simulink model "HVDC_VSC_1CPUcore_dcpl"  (Simulink 8.4)
settings: Solver=ode3  SolverMode=SingleTasking  StartTime=0.0  StopTime=70.0  FixedStep=Ts_Power  RelTol=1e-3  AbsTol=1e-2
PreLoadFcn:
  | Ts_Power=50e-6; Ts_Control=1*Ts_Power; init_cosim_IA; startup_transients_hvdc_vsc;
PostLoadFcn:
  | Ts_Power=50e-6; Ts_Control=1*Ts_Power; init_cosim_IA; startup_transients_hvdc_vsc;
InitFcn:
  | Ts_Power=50e-6; Ts_Control=1*Ts_Power; init_cosim_IA; startup_transients_hvdc_vsc;
values from neighbouring files (symbols this model uses):
  dPref1_2 = 0.125    [startup_transients_hvdc_vsc.m]
  dPref1_2_rlimit = 0.6    [startup_transients_hvdc_vsc.m]
  t_deblock_Pref1 = 0.5    [startup_transients_hvdc_vsc.m]
  t_deblock_Udref2 = 0.3    [startup_transients_hvdc_vsc.m]
  t_dPref1_2 = 25.0    (= 25)    [startup_transients_hvdc_vsc.m]
  t_SwitchITMIdc = 0.2    [startup_transients_hvdc_vsc.m]
  t_SwitchITMVdc = 0.1    [startup_transients_hvdc_vsc.m]
undefined symbols (not defined in the file or in its folder): CLARK, D1, Delta, gcbh, h, intfDelay, level, lib_mesures, magnitude, ResistanceM, rte_drive_private_lib, rte_tsb3level_hiz_rect_cb, sps_rtmsupport, Ts_intf, TSB3_hiZR
libraries: powerlib x183, spsVIMeasurementModel x102, powerlib_extras x71, powerlib_meascontrol x50, rteventslib x26, op_dpl_lib x20, rtlab x12, sps_avr x6, artemis x1
(part 6 of 13)

== system HVDC_VSC_1CPUcore_dcpl/SM_HVDC_VSC/37.5-km  cable1/Artemis DPL2 ==
  hi : Inport
  GroundI_0_1 : powerlib/Elements/Ground  LConnTagsString=a
  GroundR_0_1 : powerlib/Elements/Ground  LConnTagsString=a
  ISource_0_1 : powerlib/Electrical Sources/Controlled Current Source  Initialize=off  Source_Type=AC  Amplitude=0  Phase=0  Frequency=0  Measurements=None
  R_0_1 : powerlib/Elements/Series RLC Branch  LConnTagsString=__new0  RConnTagsString=__new0  BranchType=R  Resistance=ResistanceM(1,1)  Inductance=1.0  SetiL0=off  InitialCurrent=0  Capacitance=1.0  Setx0=off  InitialVoltage=0  Measurements=None
  VMeasure_0_1 : powerlib/Measurements/Voltage Measurement  PhasorSimulation=off  OutputType=Complex  PSBequivalent=0
  separated_model1 : op_dpl_lib/separated_model1  nphase=Phases  f=Frequency  ri=Resistance  li=Inductance  ci=Capacitance  long=Length  V1_init=[0 zeros(1,Phases); 0.1 zeros(1,Phases)]  V2_init=[0 zeros(1,Phases); 0.1 zeros(1,Phases)]  I1_init=[0 zeros(1,Phases); 0.1 zeros(1,Phases)]  I2_init=[0 zeros(1,Phases); 0.1 zeros(1,Phases)]  time_init=0.000622095723695317
  PM1 : PMIOPort  Port=1  Side=Left
  ho : Outport
  wires:
  [ho] -> ho/1
  hi/1 -> [hi]
  [V_A_1] -> separated_model1/1
  separated_model1/1 -> [I_A_1]
  [hi] -> separated_model1/2
  separated_model1/2 -> [ho]
  [I_A_1] -> ISource_0_1/1
  VMeasure_0_1/1 -> [V_A_1]
  connections:
  VMeasure_0_1/LConn1 -- ISource_0_1/RConn1 -- R_0_1/LConn1 -- PM1/RConn1
  VMeasure_0_1/LConn2 -- GroundI_0_1/LConn1 -- ISource_0_1/LConn1
  R_0_1/RConn1 -- GroundR_0_1/LConn1

== system HVDC_VSC_1CPUcore_dcpl/SM_HVDC_VSC/37.5-km  cable1/BI ==

== system HVDC_VSC_1CPUcore_dcpl/SM_HVDC_VSC/37.5-km cable/Artemis DPL1 ==
  hi : Inport
  GroundI_0_1 : powerlib/Elements/Ground  LConnTagsString=a
  GroundR_0_1 : powerlib/Elements/Ground  LConnTagsString=a
  ISource_0_1 : powerlib/Electrical Sources/Controlled Current Source  Initialize=off  Source_Type=AC  Amplitude=0  Phase=0  Frequency=0  Measurements=None
  R_0_1 : powerlib/Elements/Series RLC Branch  LConnTagsString=__new0  RConnTagsString=__new0  BranchType=R  Resistance=ResistanceM(1,1)  Inductance=1.0  SetiL0=off  InitialCurrent=0  Capacitance=1.0  Setx0=off  InitialVoltage=0  Measurements=None
  VMeasure_0_1 : powerlib/Measurements/Voltage Measurement  PhasorSimulation=off  OutputType=Complex  PSBequivalent=0
  separated_model1 : op_dpl_lib/separated_model1  nphase=Phases  f=Frequency  ri=Resistance  li=Inductance  ci=Capacitance  long=Length  V1_init=[0 zeros(1,Phases); 0.1 zeros(1,Phases)]  V2_init=[0 zeros(1,Phases); 0.1 zeros(1,Phases)]  I1_init=[0 zeros(1,Phases); 0.1 zeros(1,Phases)]  I2_init=[0 zeros(1,Phases); 0.1 zeros(1,Phases)]  time_init=0.000622095723695317
  PM1 : PMIOPort  Port=1  Side=Left
  ho : Outport
  wires:
  [ho] -> ho/1
  hi/1 -> [hi]
  [V_A_1] -> separated_model1/1
  separated_model1/1 -> [I_A_1]
  [hi] -> separated_model1/2
  separated_model1/2 -> [ho]
  [I_A_1] -> ISource_0_1/1
  VMeasure_0_1/1 -> [V_A_1]
  connections:
  VMeasure_0_1/LConn1 -- ISource_0_1/RConn1 -- R_0_1/LConn1 -- PM1/RConn1
  VMeasure_0_1/LConn2 -- GroundI_0_1/LConn1 -- ISource_0_1/LConn1
  R_0_1/RConn1 -- GroundR_0_1/LConn1

== system HVDC_VSC_1CPUcore_dcpl/SM_HVDC_VSC/37.5-km cable/Artemis DPL2 ==
  hi : Inport
  GroundI_0_1 : powerlib/Elements/Ground  LConnTagsString=a
  GroundR_0_1 : powerlib/Elements/Ground  LConnTagsString=a
  ISource_0_1 : powerlib/Electrical Sources/Controlled Current Source  Initialize=off  Source_Type=AC  Amplitude=0  Phase=0  Frequency=0  Measurements=None
  R_0_1 : powerlib/Elements/Series RLC Branch  LConnTagsString=__new0  RConnTagsString=__new0  BranchType=R  Resistance=ResistanceM(1,1)  Inductance=1.0  SetiL0=off  InitialCurrent=0  Capacitance=1.0  Setx0=off  InitialVoltage=0  Measurements=None
  VMeasure_0_1 : powerlib/Measurements/Voltage Measurement  PhasorSimulation=off  OutputType=Complex  PSBequivalent=0
  separated_model1 : op_dpl_lib/separated_model1  nphase=Phases  f=Frequency  ri=Resistance  li=Inductance  ci=Capacitance  long=Length  V1_init=[0 zeros(1,Phases); 0.1 zeros(1,Phases)]  V2_init=[0 zeros(1,Phases); 0.1 zeros(1,Phases)]  I1_init=[0 zeros(1,Phases); 0.1 zeros(1,Phases)]  I2_init=[0 zeros(1,Phases); 0.1 zeros(1,Phases)]  time_init=0.000622095723695317
  PM1 : PMIOPort  Port=1  Side=Left
  ho : Outport
  wires:
  [ho] -> ho/1
  hi/1 -> [hi]
  [V_A_1] -> separated_model1/1
  separated_model1/1 -> [I_A_1]
  [hi] -> separated_model1/2
  separated_model1/2 -> [ho]
  [I_A_1] -> ISource_0_1/1
  VMeasure_0_1/1 -> [V_A_1]
  connections:
  VMeasure_0_1/LConn1 -- ISource_0_1/RConn1 -- R_0_1/LConn1 -- PM1/RConn1
  VMeasure_0_1/LConn2 -- GroundI_0_1/LConn1 -- ISource_0_1/LConn1
  R_0_1/RConn1 -- GroundR_0_1/LConn1

== system HVDC_VSC_1CPUcore_dcpl/SM_HVDC_VSC/37.5-km cable/BI ==

== system HVDC_VSC_1CPUcore_dcpl/SM_HVDC_VSC/37.5-km cable1/Artemis DPL1 ==
  hi : Inport
  GroundI_0_1 : powerlib/Elements/Ground  LConnTagsString=a
  GroundR_0_1 : powerlib/Elements/Ground  LConnTagsString=a
  ISource_0_1 : powerlib/Electrical Sources/Controlled Current Source  Initialize=off  Source_Type=AC  Amplitude=0  Phase=0  Frequency=0  Measurements=None
  R_0_1 : powerlib/Elements/Series RLC Branch  LConnTagsString=__new0  RConnTagsString=__new0  BranchType=R  Resistance=ResistanceM(1,1)  Inductance=1.0  SetiL0=off  InitialCurrent=0  Capacitance=1.0  Setx0=off  InitialVoltage=0  Measurements=None
  VMeasure_0_1 : powerlib/Measurements/Voltage Measurement  PhasorSimulation=off  OutputType=Complex  PSBequivalent=0
  separated_model1 : op_dpl_lib/separated_model1  nphase=Phases  f=Frequency  ri=Resistance  li=Inductance  ci=Capacitance  long=Length  V1_init=[0 zeros(1,Phases); 0.1 zeros(1,Phases)]  V2_init=[0 zeros(1,Phases); 0.1 zeros(1,Phases)]  I1_init=[0 zeros(1,Phases); 0.1 zeros(1,Phases)]  I2_init=[0 zeros(1,Phases); 0.1 zeros(1,Phases)]  time_init=0.000622095723695317
  PM1 : PMIOPort  Port=1  Side=Left
  ho : Outport
  wires:
  VMeasure_0_1/1 -> [V_A_1]
  [I_A_1] -> ISource_0_1/1
  separated_model1/2 -> [ho]
  [hi] -> separated_model1/2
  separated_model1/1 -> [I_A_1]
  [V_A_1] -> separated_model1/1
  hi/1 -> [hi]
  [ho] -> ho/1
  connections:
  R_0_1/RConn1 -- GroundR_0_1/LConn1
  ISource_0_1/LConn1 -- GroundI_0_1/LConn1 -- VMeasure_0_1/LConn2
  PM1/RConn1 -- R_0_1/LConn1 -- ISource_0_1/RConn1 -- VMeasure_0_1/LConn1

== system HVDC_VSC_1CPUcore_dcpl/SM_HVDC_VSC/37.5-km cable1/Artemis DPL2 ==
  hi : Inport
  GroundI_0_1 : powerlib/Elements/Ground  LConnTagsString=a
  GroundR_0_1 : powerlib/Elements/Ground  LConnTagsString=a
  ISource_0_1 : powerlib/Electrical Sources/Controlled Current Source  Initialize=off  Source_Type=AC  Amplitude=0  Phase=0  Frequency=0  Measurements=None
  R_0_1 : powerlib/Elements/Series RLC Branch  LConnTagsString=__new0  RConnTagsString=__new0  BranchType=R  Resistance=ResistanceM(1,1)  Inductance=1.0  SetiL0=off  InitialCurrent=0  Capacitance=1.0  Setx0=off  InitialVoltage=0  Measurements=None
  VMeasure_0_1 : powerlib/Measurements/Voltage Measurement  PhasorSimulation=off  OutputType=Complex  PSBequivalent=0
  separated_model1 : op_dpl_lib/separated_model1  nphase=Phases  f=Frequency  ri=Resistance  li=Inductance  ci=Capacitance  long=Length  V1_init=[0 zeros(1,Phases); 0.1 zeros(1,Phases)]  V2_init=[0 zeros(1,Phases); 0.1 zeros(1,Phases)]  I1_init=[0 zeros(1,Phases); 0.1 zeros(1,Phases)]  I2_init=[0 zeros(1,Phases); 0.1 zeros(1,Phases)]  time_init=0.000622095723695317
  PM1 : PMIOPort  Port=1  Side=Left
  ho : Outport
  wires:
  VMeasure_0_1/1 -> [V_A_1]
  [I_A_1] -> ISource_0_1/1
  separated_model1/2 -> [ho]
  [hi] -> separated_model1/2
  separated_model1/1 -> [I_A_1]
  [V_A_1] -> separated_model1/1
  hi/1 -> [hi]
  [ho] -> ho/1
  connections:
  R_0_1/RConn1 -- GroundR_0_1/LConn1
  ISource_0_1/LConn1 -- GroundI_0_1/LConn1 -- VMeasure_0_1/LConn2
  PM1/RConn1 -- R_0_1/LConn1 -- ISource_0_1/RConn1 -- VMeasure_0_1/LConn1

== system HVDC_VSC_1CPUcore_dcpl/SM_HVDC_VSC/37.5-km cable1/BI ==

== system HVDC_VSC_1CPUcore_dcpl/SM_HVDC_VSC/Station 1 (Rectifier)/Bconv1 ==
  Kv : Gain  Gain=Ki  SaturateOnIntegerOverflow=on  OutDataTypeStr=Inherit: Same as input  ParamDataTypeStr=Inherit: Same as input
  Kv1 : Gain  Gain=Kv  SaturateOnIntegerOverflow=on  OutDataTypeStr=Inherit: Same as input  ParamDataTypeStr=Inherit: Same as input
  Mode I : spsVIMeasurementModel/Complex
  Mode V : spsVIMeasurementModel/Complex
  Model : spsVIMeasurementModel/VI  SystemSampleTime=-1
  A : PMIOPort  Port=1  Side=Left
  B : PMIOPort  Port=2  Side=Left
  C : PMIOPort  Port=3  Side=Left
  a : PMIOPort  Port=4  Side=Right
  b : PMIOPort  Port=5  Side=Right
  c : PMIOPort  Port=6  Side=Right
  tag scope: Iv_abc1=global, Uv_abc1=global
  wires:
  Model/2 -> Kv/1
  Model/1 -> Kv1/1
  Kv/1 -> Mode I/1
  Kv1/1 -> Mode V/1
  Mode I/1 -> [Iv_abc1]
  Mode V/1 -> [Uv_abc1]
  connections:
  Model/RConn3 -- c/RConn1
  Model/RConn1 -- a/RConn1
  Model/RConn2 -- b/RConn1
  Model/LConn3 -- C/RConn1
  Model/LConn1 -- A/RConn1
  Model/LConn2 -- B/RConn1

== system HVDC_VSC_1CPUcore_dcpl/SM_HVDC_VSC/Station 1 (Rectifier)/Bfilter1 ==
  Iabc : Terminator
  Kv : Gain  Gain=Ki  SaturateOnIntegerOverflow=on  OutDataTypeStr=Inherit: Same as input  ParamDataTypeStr=Inherit: Same as input
  Kv1 : Gain  Gain=Kv  SaturateOnIntegerOverflow=on  OutDataTypeStr=Inherit: Same as input  ParamDataTypeStr=Inherit: Same as input
  Mode I : spsVIMeasurementModel/Complex
  Mode V : spsVIMeasurementModel/Complex
  Model : spsVIMeasurementModel/V  SystemSampleTime=-1
  A : PMIOPort  Port=1  Side=Left
  B : PMIOPort  Port=2  Side=Left
  C : PMIOPort  Port=3  Side=Left
  a : PMIOPort  Port=4  Side=Right
  b : PMIOPort  Port=5  Side=Right
  c : PMIOPort  Port=6  Side=Right
  tag scope: Uf_abc1=global
  wires:
  Model/2 -> Kv/1
  Model/1 -> Kv1/1
  Kv/1 -> Mode I/1
  Kv1/1 -> Mode V/1
  Mode I/1 -> Iabc/1
  Mode V/1 -> [Uf_abc1]
  connections:
  Model/RConn3 -- c/RConn1
  Model/RConn1 -- a/RConn1
  Model/RConn2 -- b/RConn1
  Model/LConn3 -- C/RConn1
  Model/LConn1 -- A/RConn1
  Model/LConn2 -- B/RConn1

== system HVDC_VSC_1CPUcore_dcpl/SM_HVDC_VSC/Station 1 (Rectifier)/Filters 60Hz2 ==
  note: High-pass
      | damped filters
  note: AC Filters, 40 Mvar @ 100 kV
  "27th 18 Mvar Q = 15 " : powerlib/Elements/Three-Phase Harmonic Filter  LConnTagsString=A|B|C  FilterType=High-pass  FilterConnection=Y (grounded)  ParNom="[100e3  60]"  Qc=80e6 * 0.45  Fr=27*60  Frd=[11*60 13*60]  Q=15  Measurements=None
      settings: AttributesFormatString=\n
  "54th 22 Mvar Q = 15 " : powerlib/Elements/Three-Phase Harmonic Filter  LConnTagsString=A|B|C  FilterType=High-pass  FilterConnection=Y (grounded)  ParNom="[100e3  60]"  Qc=80e6 * 0.55  Fr=(2*27)*60  Frd=[11*60 13*60]  Q=15  Measurements=None
      settings: AttributesFormatString=\n
  A : PMIOPort  Port=1  Side=Left
  B : PMIOPort  Port=2  Side=Left
  C : PMIOPort  Port=3  Side=Left
  connections:
  "54th 22 Mvar Q = 15 "/LConn3 -- C/RConn1 -- "27th 18 Mvar Q = 15 "/LConn3
  "54th 22 Mvar Q = 15 "/LConn2 -- B/RConn1 -- "27th 18 Mvar Q = 15 "/LConn2
  "54th 22 Mvar Q = 15 "/LConn1 -- A/RConn1 -- "27th 18 Mvar Q = 15 "/LConn1

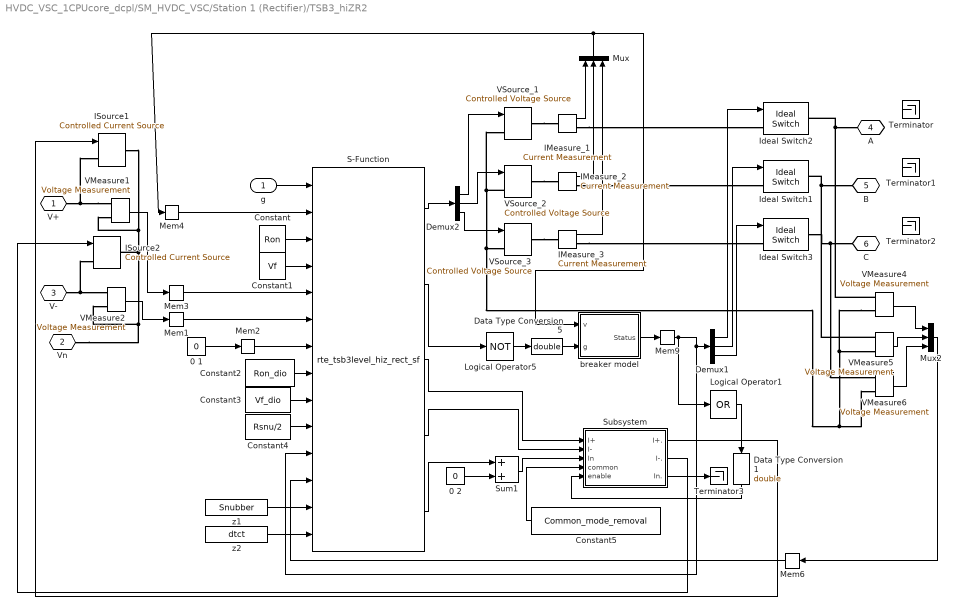
== system HVDC_VSC_1CPUcore_dcpl/SM_HVDC_VSC/Station 1 (Rectifier)/TSB3_hiZR2 ==
  g : Inport
  0 1 : Constant  Value=0
  0 2 : Constant  Value=0
  Constant : Constant  Value=Ron
  Constant1 : Constant  Value=Vf
  Constant2 : Constant  Value=Ron_dio
  Constant3 : Constant  Value=Vf_dio
  Constant4 : Constant  Value=Rsnu/2
  Constant5 : Constant  Value=Common_mode_removal
  Data Type Conversion1 : DataTypeConversion  OutDataTypeStr=double  SaturateOnIntegerOverflow=on  RndMeth=Zero
  Data Type Conversion5 : DataTypeConversion  OutDataTypeStr=double  SaturateOnIntegerOverflow=on  RndMeth=Zero
  Demux1 : Demux  Outputs=3
  Demux2 : Demux  Outputs=3
  IMeasure_1 : powerlib/Measurements/Current Measurement  PhasorSimulation=off  OutputType=Magnitude  PSBequivalent=0
  IMeasure_2 : powerlib/Measurements/Current Measurement  PhasorSimulation=off  OutputType=Magnitude  PSBequivalent=0
  IMeasure_3 : powerlib/Measurements/Current Measurement  PhasorSimulation=off  OutputType=Magnitude  PSBequivalent=0
  ISource1 : powerlib/Electrical Sources/Controlled Current Source  Initialize=off  Source_Type=AC  Amplitude=0  Phase=0  Frequency=0  Measurements=None
  ISource2 : powerlib/Electrical Sources/Controlled Current Source  Initialize=off  Source_Type=AC  Amplitude=0  Phase=0  Frequency=0  Measurements=None
  Ideal Switch1 : powerlib/Power Electronics/Ideal Switch  Ron=0.00001  Lon=0  IC=0  Rs=Rhi  Cs=inf  Measurements=off
  Ideal Switch2 : powerlib/Power Electronics/Ideal Switch  Ron=0.00001  Lon=0  IC=0  Rs=Rhi  Cs=inf  Measurements=off
  Ideal Switch3 : powerlib/Power Electronics/Ideal Switch  Ron=0.00001  Lon=0  IC=0  Rs=Rhi  Cs=inf  Measurements=off
  Logical Operator1 : Logic  Operator=OR  Inputs=1  AllPortsSameDT=off  OutDataTypeStr=boolean
  Logical Operator5 : Logic  Operator=NOT  Inputs=1  AllPortsSameDT=off  OutDataTypeStr=boolean
  Mem{1..4,6,9} (6 alike) : Memory  InheritSampleTime=on
  Mux : Mux  Inputs=3
  Mux2 : Mux  Inputs=3
  S-Function : S-Function  FunctionName=rte_tsb3level_hiz_rect_sf  EnableBusSupport=off
  Subsystem : Subsystem
  Sum1 : Sum  Inputs=2  SaturateOnIntegerOverflow=on  InputSameDT=on  OutDataTypeStr=Inherit: Same as first input
  Terminator{,1..3} (4 alike) : Terminator
  VMeasure{1..2,4..6} (5 alike) : powerlib/Measurements/Voltage Measurement  PhasorSimulation=off  OutputType=Magnitude  PSBequivalent=0
  VSource_1 : powerlib/Electrical Sources/Controlled Voltage Source  Initialize=off  Source_Type=AC  Amplitude=0  Phase=0  Frequency=0  Measurements=None
  VSource_2 : powerlib/Electrical Sources/Controlled Voltage Source  Initialize=off  Source_Type=AC  Amplitude=0  Phase=0  Frequency=0  Measurements=None
  VSource_3 : powerlib/Electrical Sources/Controlled Voltage Source  Initialize=off  Source_Type=AC  Amplitude=0  Phase=0  Frequency=0  Measurements=None
  breaker model : Subsystem
  z1 : Constant  Value=Snubber
  z2 : Constant  Value=dtct
  V+ : PMIOPort  Port=1  Side=Left
  Vn : PMIOPort  Port=2  Side=Left
  V- : PMIOPort  Port=3  Side=Left
  A : PMIOPort  Port=4  Side=Right
  B : PMIOPort  Port=5  Side=Right
  C : PMIOPort  Port=6  Side=Right
  wires:
  z1/1 -> S-Function/13
  Constant3/1 -> S-Function/9
  Constant2/1 -> S-Function/8
  S-Function/5 -> Sum1/1
  S-Function/4 -> Subsystem/2(I-)
  S-Function/3 -> Subsystem/1(I+)
  VMeasure2/1 -> Mem1/1
  VMeasure1/1 -> Mem3/1
  Constant1/1 -> S-Function/4
  Constant/1 -> S-Function/3
  S-Function/2 -> Logical Operator5/1
  Mux/1 -> Mem4/1, breaker model/1(v)
  Demux1/3 -> Ideal Switch3/1
  Demux1/2 -> Ideal Switch1/1
  Demux1/1 -> Ideal Switch2/1
  Mem4/1 -> S-Function/2
  Mem3/1 -> S-Function/5
  Mem1/1 -> S-Function/6
  g/1 -> S-Function/1
  IMeasure_3/1 -> Mux/3
  IMeasure_2/1 -> Mux/2
  IMeasure_1/1 -> Mux/1
  Constant4/1 -> S-Function/10
  VMeasure4/1 -> Mux2/1
  VMeasure5/1 -> Mux2/2
  Mux2/1 -> Mem6/1
  VMeasure6/1 -> Mux2/3
  Mem6/1 -> S-Function/12
  Subsystem/1(I+.) -> ISource1/1
  Subsystem/2(I-.) -> ISource2/1
  Sum1/1 -> Subsystem/3(In)
  Constant5/1 -> Subsystem/4(common)
  Data Type Conversion5/1 -> breaker model/2(g)
  breaker model/1(Status) -> Mem9/1
  Logical Operator5/1 -> Data Type Conversion5/1
  Mem9/1 -> S-Function/11, Demux1/1, Logical Operator1/1
  Logical Operator1/1 -> Data Type Conversion1/1
  Data Type Conversion1/1 -> Subsystem/5(enable)
  S-Function/1 -> Demux2/1
  Demux2/1 -> VSource_1/1
  Demux2/2 -> VSource_2/1
  Demux2/3 -> VSource_3/1
  Mem2/1 -> S-Function/7
  ? -> Terminator/1
  ? -> Terminator1/1
  z2/1 -> S-Function/14
  ? -> Terminator2/1
  0 1/1 -> Mem2/1
  0 2/1 -> Sum1/2
  Subsystem/3(In.) -> Terminator3/1
  connections:
  VMeasure2/LConn2 -- Vn/RConn1 -- ISource1/RConn1 -- VMeasure1/LConn2 -- ISource2/RConn1
  IMeasure_3/RConn1 -- Ideal Switch3/LConn1
  IMeasure_2/RConn1 -- Ideal Switch1/LConn1
  IMeasure_1/RConn1 -- Ideal Switch2/LConn1
  VMeasure5/LConn1 -- Ideal Switch1/RConn1 -- B/RConn1
  VMeasure1/LConn1 -- ISource1/LConn1 -- V+/RConn1
  VSource_3/RConn1 -- IMeasure_3/LConn1
  VSource_2/RConn1 -- IMeasure_2/LConn1
  VSource_1/RConn1 -- IMeasure_1/LConn1
  VMeasure4/LConn2 -- VMeasure5/LConn2 -- VSource_1/LConn1 -- VSource_2/LConn1 -- VSource_3/LConn1 -- VMeasure6/LConn2
  VMeasure4/LConn1 -- Ideal Switch2/RConn1 -- A/RConn1
  Ideal Switch3/RConn1 -- VMeasure6/LConn1 -- C/RConn1
  V-/RConn1 -- ISource2/LConn1 -- VMeasure2/LConn1

== system HVDC_VSC_1CPUcore_dcpl/SM_HVDC_VSC/Station 2 (Inverter)/Bconv2 ==
  Kv : Gain  Gain=Ki  SaturateOnIntegerOverflow=on  OutDataTypeStr=Inherit: Same as input  ParamDataTypeStr=Inherit: Same as input
  Kv1 : Gain  Gain=Kv  SaturateOnIntegerOverflow=on  OutDataTypeStr=Inherit: Same as input  ParamDataTypeStr=Inherit: Same as input
  Mode I : spsVIMeasurementModel/Complex
  Mode V : spsVIMeasurementModel/Complex
  Model : spsVIMeasurementModel/VI  SystemSampleTime=-1
  A : PMIOPort  Port=1  Side=Left
  B : PMIOPort  Port=2  Side=Left
  C : PMIOPort  Port=3  Side=Left
  a : PMIOPort  Port=4  Side=Right
  b : PMIOPort  Port=5  Side=Right
  c : PMIOPort  Port=6  Side=Right
  tag scope: Iv_abc2=global, Uv_abc2=global
  wires:
  Model/2 -> Kv/1
  Model/1 -> Kv1/1
  Kv/1 -> Mode I/1
  Kv1/1 -> Mode V/1
  Mode I/1 -> [Iv_abc2]
  Mode V/1 -> [Uv_abc2]
  connections:
  Model/RConn3 -- c/RConn1
  Model/RConn1 -- a/RConn1
  Model/RConn2 -- b/RConn1
  Model/LConn3 -- C/RConn1
  Model/LConn1 -- A/RConn1
  Model/LConn2 -- B/RConn1

== system HVDC_VSC_1CPUcore_dcpl/SM_HVDC_VSC/Station 2 (Inverter)/Bfilter2 ==
  Iabc : Terminator
  Kv : Gain  Gain=Ki  SaturateOnIntegerOverflow=on  OutDataTypeStr=Inherit: Same as input  ParamDataTypeStr=Inherit: Same as input
  Kv1 : Gain  Gain=Kv  SaturateOnIntegerOverflow=on  OutDataTypeStr=Inherit: Same as input  ParamDataTypeStr=Inherit: Same as input
  Mode I : spsVIMeasurementModel/Complex
  Mode V : spsVIMeasurementModel/Complex
  Model : spsVIMeasurementModel/V  SystemSampleTime=-1
  A : PMIOPort  Port=1  Side=Left
  B : PMIOPort  Port=2  Side=Left
  C : PMIOPort  Port=3  Side=Left
  a : PMIOPort  Port=4  Side=Right
  b : PMIOPort  Port=5  Side=Right
  c : PMIOPort  Port=6  Side=Right
  tag scope: Uf_abc2=global
  wires:
  Model/2 -> Kv/1
  Model/1 -> Kv1/1
  Kv/1 -> Mode I/1
  Kv1/1 -> Mode V/1
  Mode I/1 -> Iabc/1
  Mode V/1 -> [Uf_abc2]
  connections:
  Model/RConn3 -- c/RConn1
  Model/RConn1 -- a/RConn1
  Model/RConn2 -- b/RConn1
  Model/LConn3 -- C/RConn1
  Model/LConn1 -- A/RConn1
  Model/LConn2 -- B/RConn1

== system HVDC_VSC_1CPUcore_dcpl/SM_HVDC_VSC/Station 2 (Inverter)/Filters 60Hz2 ==
  note: High-pass
      | damped filters
  note: AC Filters, 40 Mvar @ 100 kV
  "27th 18 Mvar Q = 15 " : powerlib/Elements/Three-Phase Harmonic Filter  LConnTagsString=A|B|C  FilterType=High-pass  FilterConnection=Y (grounded)  ParNom="[100e3  60]"  Qc=80e6 * 0.45  Fr=27*60  Frd=[11*60 13*60]  Q=15  Measurements=None
      settings: AttributesFormatString=\n
  "54th 22 Mvar Q = 15 " : powerlib/Elements/Three-Phase Harmonic Filter  LConnTagsString=A|B|C  FilterType=High-pass  FilterConnection=Y (grounded)  ParNom="[100e3  60]"  Qc=80e6 * 0.55  Fr=(2*27)*60  Frd=[11*60 13*60]  Q=15  Measurements=None
      settings: AttributesFormatString=\n
  A : PMIOPort  Port=1  Side=Left
  B : PMIOPort  Port=2  Side=Left
  C : PMIOPort  Port=3  Side=Left
  connections:
  "27th 18 Mvar Q = 15 "/LConn3 -- "54th 22 Mvar Q = 15 "/LConn3 -- C/RConn1
  "27th 18 Mvar Q = 15 "/LConn2 -- "54th 22 Mvar Q = 15 "/LConn2 -- B/RConn1
  "27th 18 Mvar Q = 15 "/LConn1 -- "54th 22 Mvar Q = 15 "/LConn1 -- A/RConn1

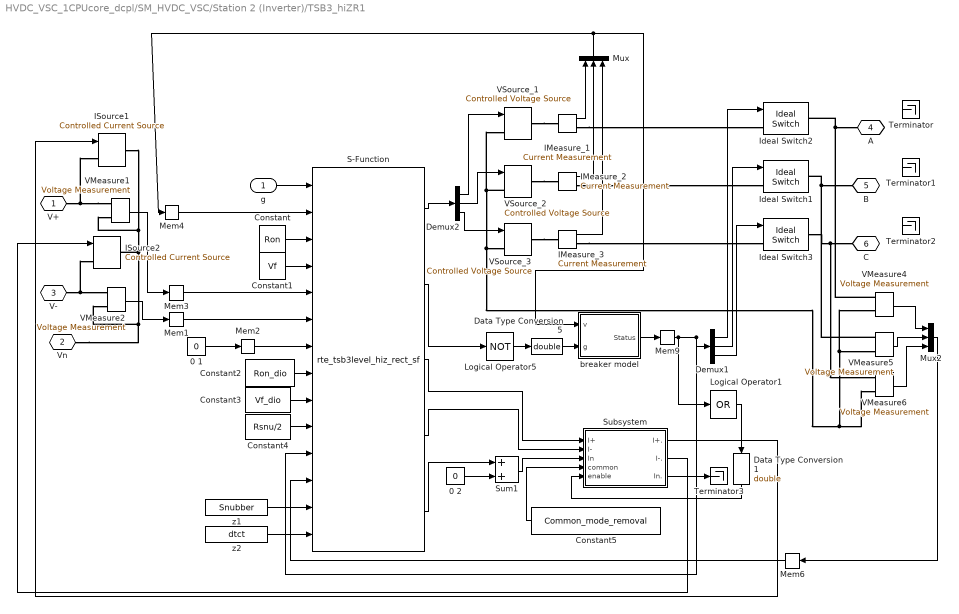
== system HVDC_VSC_1CPUcore_dcpl/SM_HVDC_VSC/Station 2 (Inverter)/TSB3_hiZR1 ==
  g : Inport
  0 1 : Constant  Value=0
  0 2 : Constant  Value=0
  Constant : Constant  Value=Ron
  Constant1 : Constant  Value=Vf
  Constant2 : Constant  Value=Ron_dio
  Constant3 : Constant  Value=Vf_dio
  Constant4 : Constant  Value=Rsnu/2
  Constant5 : Constant  Value=Common_mode_removal
  Data Type Conversion1 : DataTypeConversion  OutDataTypeStr=double  SaturateOnIntegerOverflow=on  RndMeth=Zero
  Data Type Conversion5 : DataTypeConversion  OutDataTypeStr=double  SaturateOnIntegerOverflow=on  RndMeth=Zero
  Demux1 : Demux  Outputs=3
  Demux2 : Demux  Outputs=3
  IMeasure_1 : powerlib/Measurements/Current Measurement  PhasorSimulation=off  OutputType=Magnitude  PSBequivalent=0
  IMeasure_2 : powerlib/Measurements/Current Measurement  PhasorSimulation=off  OutputType=Magnitude  PSBequivalent=0
  IMeasure_3 : powerlib/Measurements/Current Measurement  PhasorSimulation=off  OutputType=Magnitude  PSBequivalent=0
  ISource1 : powerlib/Electrical Sources/Controlled Current Source  Initialize=off  Source_Type=AC  Amplitude=0  Phase=0  Frequency=0  Measurements=None
  ISource2 : powerlib/Electrical Sources/Controlled Current Source  Initialize=off  Source_Type=AC  Amplitude=0  Phase=0  Frequency=0  Measurements=None
  Ideal Switch1 : powerlib/Power Electronics/Ideal Switch  Ron=0.00001  Lon=0  IC=0  Rs=Rhi  Cs=inf  Measurements=off
  Ideal Switch2 : powerlib/Power Electronics/Ideal Switch  Ron=0.00001  Lon=0  IC=0  Rs=Rhi  Cs=inf  Measurements=off
  Ideal Switch3 : powerlib/Power Electronics/Ideal Switch  Ron=0.00001  Lon=0  IC=0  Rs=Rhi  Cs=inf  Measurements=off
  Logical Operator1 : Logic  Operator=OR  Inputs=1  AllPortsSameDT=off  OutDataTypeStr=boolean
  Logical Operator5 : Logic  Operator=NOT  Inputs=1  AllPortsSameDT=off  OutDataTypeStr=boolean
  Mem{1..4,6,9} (6 alike) : Memory  InheritSampleTime=on
  Mux : Mux  Inputs=3
  Mux2 : Mux  Inputs=3
  S-Function : S-Function  FunctionName=rte_tsb3level_hiz_rect_sf  EnableBusSupport=off
  Subsystem : Subsystem
  Sum1 : Sum  Inputs=2  SaturateOnIntegerOverflow=on  InputSameDT=on  OutDataTypeStr=Inherit: Same as first input
  Terminator{,1..3} (4 alike) : Terminator
  VMeasure{1..2,4..6} (5 alike) : powerlib/Measurements/Voltage Measurement  PhasorSimulation=off  OutputType=Magnitude  PSBequivalent=0
  VSource_1 : powerlib/Electrical Sources/Controlled Voltage Source  Initialize=off  Source_Type=AC  Amplitude=0  Phase=0  Frequency=0  Measurements=None
  VSource_2 : powerlib/Electrical Sources/Controlled Voltage Source  Initialize=off  Source_Type=AC  Amplitude=0  Phase=0  Frequency=0  Measurements=None
  VSource_3 : powerlib/Electrical Sources/Controlled Voltage Source  Initialize=off  Source_Type=AC  Amplitude=0  Phase=0  Frequency=0  Measurements=None
  breaker model : Subsystem
  z1 : Constant  Value=Snubber
  z2 : Constant  Value=dtct
  V+ : PMIOPort  Port=1  Side=Left
  Vn : PMIOPort  Port=2  Side=Left
  V- : PMIOPort  Port=3  Side=Left
  A : PMIOPort  Port=4  Side=Right
  B : PMIOPort  Port=5  Side=Right
  C : PMIOPort  Port=6  Side=Right
  wires:
  z1/1 -> S-Function/13
  Constant3/1 -> S-Function/9
  Constant2/1 -> S-Function/8
  S-Function/5 -> Sum1/1
  S-Function/4 -> Subsystem/2(I-)
  S-Function/3 -> Subsystem/1(I+)
  VMeasure2/1 -> Mem1/1
  VMeasure1/1 -> Mem3/1
  Constant1/1 -> S-Function/4
  Constant/1 -> S-Function/3
  S-Function/2 -> Logical Operator5/1
  Mux/1 -> Mem4/1, breaker model/1(v)
  Demux1/3 -> Ideal Switch3/1
  Demux1/2 -> Ideal Switch1/1
  Demux1/1 -> Ideal Switch2/1
  Mem4/1 -> S-Function/2
  Mem3/1 -> S-Function/5
  Mem1/1 -> S-Function/6
  g/1 -> S-Function/1
  IMeasure_3/1 -> Mux/3
  IMeasure_2/1 -> Mux/2
  IMeasure_1/1 -> Mux/1
  Constant4/1 -> S-Function/10
  VMeasure4/1 -> Mux2/1
  VMeasure5/1 -> Mux2/2
  Mux2/1 -> Mem6/1
  VMeasure6/1 -> Mux2/3
  Mem6/1 -> S-Function/12
  Subsystem/1(I+.) -> ISource1/1
  Subsystem/2(I-.) -> ISource2/1
  Sum1/1 -> Subsystem/3(In)
  Constant5/1 -> Subsystem/4(common)
  Data Type Conversion5/1 -> breaker model/2(g)
  breaker model/1(Status) -> Mem9/1
  Logical Operator5/1 -> Data Type Conversion5/1
  Mem9/1 -> S-Function/11, Demux1/1, Logical Operator1/1
  Logical Operator1/1 -> Data Type Conversion1/1
  Data Type Conversion1/1 -> Subsystem/5(enable)
  S-Function/1 -> Demux2/1
  Demux2/1 -> VSource_1/1
  Demux2/2 -> VSource_2/1
  Demux2/3 -> VSource_3/1
  Mem2/1 -> S-Function/7
  ? -> Terminator/1
  ? -> Terminator1/1
  z2/1 -> S-Function/14
  ? -> Terminator2/1
  0 1/1 -> Mem2/1
  0 2/1 -> Sum1/2
  Subsystem/3(In.) -> Terminator3/1
  connections:
  Vn/RConn1 -- ISource1/RConn1 -- VMeasure1/LConn2 -- ISource2/RConn1 -- VMeasure2/LConn2
  IMeasure_3/RConn1 -- Ideal Switch3/LConn1
  IMeasure_2/RConn1 -- Ideal Switch1/LConn1
  IMeasure_1/RConn1 -- Ideal Switch2/LConn1
  VMeasure5/LConn1 -- Ideal Switch1/RConn1 -- B/RConn1
  VMeasure1/LConn1 -- ISource1/LConn1 -- V+/RConn1
  VSource_3/RConn1 -- IMeasure_3/LConn1
  VSource_2/RConn1 -- IMeasure_2/LConn1
  VSource_1/RConn1 -- IMeasure_1/LConn1
  VSource_1/LConn1 -- VSource_2/LConn1 -- VSource_3/LConn1 -- VMeasure6/LConn2 -- VMeasure4/LConn2 -- VMeasure5/LConn2
  VMeasure4/LConn1 -- Ideal Switch2/RConn1 -- A/RConn1
  Ideal Switch3/RConn1 -- VMeasure6/LConn1 -- C/RConn1
  V-/RConn1 -- ISource2/LConn1 -- VMeasure2/LConn1

== system HVDC_VSC_1CPUcore_dcpl/SM_HVDC_VSC/VSC Controller (Station 1)/3-level firing pulse unit for TSB ==
  3 phase output frequency : Inport
  wt : Inport  Port=2
  Carriers Generator : Subsystem
  Demux3 : Demux  Outputs=3
  Gain5 : Gain  SaturateOnIntegerOverflow=on  OutDataTypeStr=Inherit: Same as input  ParamDataTypeStr=Inherit: Same as input
  Gain6 : Gain  SaturateOnIntegerOverflow=on  OutDataTypeStr=Inherit: Same as input  ParamDataTypeStr=Inherit: Same as input
  Mux3 : Mux  Inputs=12
  RTE Period Meter : rteventslib/Signal Attributes/RTE Period Meter  Period=off  Frequency=off  EdgeType=Rising edges  TOn=off  TOff=off  DutyCycle=on  DuringType=Calculation step  MinimumFrequency=0
  Subsystem1 : Subsystem
  Subsystem2 : Subsystem
  Subsystem6 : Subsystem
  duty : Outport
  wires:
  Mux3/1 -> RTE Period Meter/1
  Subsystem2/4(4) -> Mux3/12
  Subsystem2/3(3) -> Mux3/11
  Subsystem2/2(2) -> Mux3/10
  Subsystem2/1(1) -> Mux3/9
  Subsystem1/4(4) -> Mux3/8
  Subsystem1/3(3) -> Mux3/7
  Subsystem1/2(2) -> Mux3/6
  Subsystem1/1(1) -> Mux3/5
  Subsystem6/4(4) -> Mux3/4
  Subsystem6/3(3) -> Mux3/3
  Subsystem6/2(2) -> Mux3/2
  Subsystem6/1(1) -> Mux3/1
  Carriers Generator/2(C-) -> Gain6/1
  Carriers Generator/1(C+) -> Gain5/1
  Gain6/1 -> Subsystem1/3(c-), Subsystem2/3(c-), Subsystem6/3(c-)
  Gain5/1 -> Subsystem1/2(c+), Subsystem2/2(c+), Subsystem6/2(c+)
  wt/1 -> Carriers Generator/1(theta)
  Demux3/1 -> Subsystem6/1(in)
  Demux3/2 -> Subsystem1/1(in)
  Demux3/3 -> Subsystem2/1(in)
  3 phase output frequency/1 -> Demux3/1
  RTE Period Meter/1 -> duty/1

== system HVDC_VSC_1CPUcore_dcpl/SM_HVDC_VSC/VSC Controller (Station 1)/Anti-aliasing Filters ==
  note: Filtering
  note: Low-pass filter
  "Uabc " : Inport  PortDimensions=3
  "Iabc " : Inport  Port=2  PortDimensions=3
  "Uf_abc  " : Inport  Port=3  PortDimensions=3
  "Iv_abc " : Inport  Port=4  PortDimensions=3
  "Udc_pn  " : Inport  Port=5
  "Idc_pn " : Inport  Port=6
  2nd-Order Filter{1..9} (9 alike) : powerlib_extras/Discrete  Control Blocks/Discrete  2nd-Order Filter  FilterType=Lowpass  Fo=f0_aa  Zeta=zeta  Ts=Ts_Control  Initialize=off  Vac_Init=[0.8 -25 60]  Vdc_Init=-0.4  PlotResponse=off  param1=[1 2000 0.2]
  2nd-Order f0_aa {,1..6} (7 alike) : powerlib_extras/Discrete  Control Blocks/Discrete  2nd-Order Filter  FilterType=Lowpass  Fo=f0_aa  Zeta=zeta  Ts=Ts_Control  Initialize=off  Vac_Init=[0.8 -25 60]  Vdc_Init=-0.4  PlotResponse=off  param1=[1 2000 0.2]
  Demux{,1..3} (4 alike) : Demux  Outputs=3
  Demux4 : Demux  Outputs=2
  Demux5 : Demux  Outputs=2
  Mux{,1..3} (4 alike) : Mux  Inputs=3
  Mux4 : Mux  Inputs=2
  Mux5 : Mux  Inputs=2
  Uabc : Outport
  Iabc : Outport  Port=2
  Uf_abc : Outport  Port=3
  " Iv_abc" : Outport  Port=4
  "Udc_pn " : Outport  Port=5
  " Idc_pn" : Outport  Port=6
  wires:
  Mux1/1 -> Uf_abc/1
  Demux1/2 -> 2nd-Order Filter4/1
  Demux1/3 -> 2nd-Order Filter5/1
  2nd-Order Filter5/1 -> Mux1/3
  2nd-Order Filter4/1 -> Mux1/2
  2nd-Order Filter3/1 -> Mux1/1
  Demux1/1 -> 2nd-Order Filter3/1
  "Uf_abc  "/1 -> Demux1/1
  Demux/2 -> 2nd-Order Filter1/1
  Demux/3 -> 2nd-Order Filter2/1
  2nd-Order Filter2/1 -> Mux/3
  2nd-Order Filter1/1 -> Mux/2
  Mux/1 -> " Iv_abc"/1
  "Iv_abc "/1 -> Demux/1
  Mux2/1 -> Uabc/1
  Demux2/2 -> 2nd-Order Filter7/1
  Demux2/3 -> 2nd-Order Filter8/1
  2nd-Order Filter8/1 -> Mux2/3
  2nd-Order Filter7/1 -> Mux2/2
  2nd-Order Filter6/1 -> Mux2/1
  Demux2/1 -> 2nd-Order Filter6/1
  "Uabc "/1 -> Demux2/1
  Mux3/1 -> Iabc/1
  Demux3/2 -> 2nd-Order f0_aa 5/1
  Demux3/3 -> 2nd-Order f0_aa 6/1
  2nd-Order f0_aa 6/1 -> Mux3/3
  2nd-Order f0_aa 5/1 -> Mux3/2
  2nd-Order f0_aa 4/1 -> Mux3/1
  Demux3/1 -> 2nd-Order f0_aa 4/1
  "Iabc "/1 -> Demux3/1
  Demux/1 -> 2nd-Order Filter9/1
  2nd-Order Filter9/1 -> Mux/1
  2nd-Order f0_aa 2/1 -> Mux4/1
  2nd-Order f0_aa 3/1 -> Mux4/2
  Mux4/1 -> " Idc_pn"/1
  "2nd-Order f0_aa "/1 -> Mux5/1
  2nd-Order f0_aa 1/1 -> Mux5/2
  Mux5/1 -> "Udc_pn "/1
  Demux4/1 -> 2nd-Order f0_aa 2/1
  Demux4/2 -> 2nd-Order f0_aa 3/1
  "Idc_pn "/1 -> Demux4/1
  Demux5/1 -> "2nd-Order f0_aa "/1
  Demux5/2 -> 2nd-Order f0_aa 1/1
  "Udc_pn  "/1 -> Demux5/1

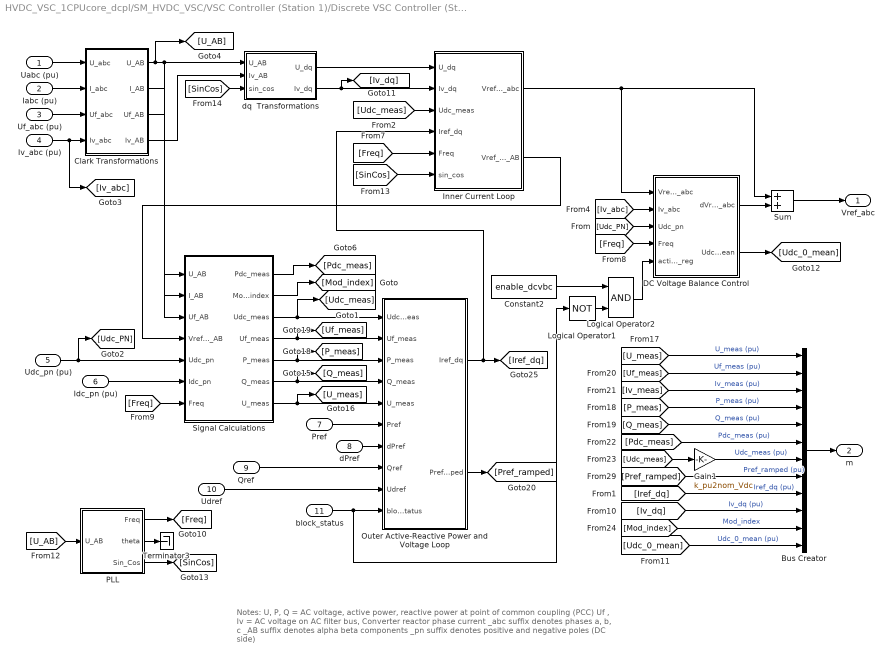
== system HVDC_VSC_1CPUcore_dcpl/SM_HVDC_VSC/VSC Controller (Station 1)/Discrete VSC Controller (Station 1) ==
  note: Notes:
      | U, P, Q = AC voltage, active power, reactive power at point of common coupling (PCC)
      | Uf , Iv  = AC voltage on AC filter bus, Converter reactor phase current
      | _abc suffix denotes phases a, b, c
      | _AB  suffix denotes alpha beta components
      | _pn  suffix denotes positive and negative poles (DC side)
  Uabc (pu) : Inport
  Iabc (pu) : Inport  Port=2
  Uf_abc (pu) : Inport  Port=3
  Iv_abc (pu) : Inport  Port=4
  Udc_pn (pu) : Inport  Port=5
  Idc_pn (pu) : Inport  Port=6
  Pref : Inport  Port=7
  dPref : Inport  Port=8
  Qref : Inport  Port=9
  Udref : Inport  Port=10
  block_status : Inport  Port=11
  Bus Creator : BusCreator  Inputs=12
  Clark Transformations : Subsystem
  Constant2 : Constant  Value=enable_dcvbc
  DC Voltage Balance Control : Subsystem
  Gain1 : Gain  Gain=k_pu2nom_Vdc  SaturateOnIntegerOverflow=on  OutDataTypeStr=Inherit: Same as input  ParamDataTypeStr=Inherit: Same as input
  Inner Current Loop : Subsystem
  Logical Operator1 : Logic  Operator=NOT  Inputs=1  AllPortsSameDT=off
  Logical Operator2 : Logic  AllPortsSameDT=off
  Outer Active-Reactive Power and Voltage Loop : Subsystem
  PLL : Subsystem  AncestorBlock=|  mask(Discrete 3-phase PLL){Fmin=f_min_pll, Par_Init=[0   60], ParK=[Kp_pll  Ki_pll], Ts=Ts_Control}
      | powerlib_extras/Discrete 
      | Control Blocks/Discrete
      | 3-phase PLL
      mask prompts: Fmin "Minimum frequency (Hz):"; Par_Init "Initial inputs:[ Phase(degrees)   Frequency(Hz) ]"; ParK "Regulator gains [ Kp  Ki ]"; Ts "Sample time:"
      mask help:
      | This Phase Locked Loop (PLL) system can be used  to synchronize on a set of variable frequency, three-phase sinusoidal signals.
      |
      | Input 1: Vector containing the normalized
      |              three-phase signals [Va Vb Vc]
      | Output 1:  Measured frequency (Hz) = w/(2pi)
      | Output 2:  Ramp w.t   varying between  0 and 2*pi,
      | synchronized on zero crossings of the fundamental (positive-sequence) of phase A.
      | Output 3: Vector [sin(wt) cos(wt)]
      mask init:
      | Kp=ParK(1);
      | Ki=ParK(2);
      | Phase_Init=Par_Init(1);
      | Finit=Par_Init(2);
  Signal Calculations : Subsystem
  Sum : Sum  SaturateOnIntegerOverflow=on
  Terminator3 : Terminator
  dq  Transformations : Subsystem
  Vref_abc : Outport
  m : Outport  Port=2
  wires:
  Outer Active-Reactive Power and Voltage Loop/1(Iref_dq) -> Inner Current Loop/4(Iref_dq), [Iref_dq]
  dq  Transformations/2(Iv_dq) -> Inner Current Loop/2(Iv_dq), [Iv_dq]
  Inner Current Loop/1(Vref_lim_abc) -> Sum/1, DC Voltage Balance Control/1(Vref_lim_abc)
  dq  Transformations/1(U_dq) -> Inner Current Loop/1(U_dq)
  Signal Calculations/3(Udc_meas) -> Outer Active-Reactive Power and Voltage Loop/1(Udc_meas), [Udc_meas]
  Signal Calculations/4(Uf_meas) -> Outer Active-Reactive Power and Voltage Loop/2(Uf_meas), [Uf_meas]
  Signal Calculations/6(Q_meas) -> Outer Active-Reactive Power and Voltage Loop/4(Q_meas), [Q_meas]
  Signal Calculations/5(P_meas) -> Outer Active-Reactive Power and Voltage Loop/3(P_meas), [P_meas]
  Clark Transformations/1(U_AB) -> dq  Transformations/1(U_AB), Signal Calculations/1(U_AB), [U_AB]
  Signal Calculations/1(Pdc_meas) -> [Pdc_meas]
  Constant2/1 -> Logical Operator2/1
  Pref/1 -> Outer Active-Reactive Power and Voltage Loop/6(Pref)
  dPref/1 -> Outer Active-Reactive Power and Voltage Loop/7(dPref)
  Qref/1 -> Outer Active-Reactive Power and Voltage Loop/8(Qref)
  PLL/2(theta) -> Terminator3/1
  Logical Operator2/1 -> DC Voltage Balance Control/5(activate_reg)
  [Udc_PN] -> DC Voltage Balance Control/3(Udc_pn)
  Udc_pn (pu)/1 -> Signal Calculations/5(Udc_pn), [Udc_PN]
  [Iv_abc] -> DC Voltage Balance Control/2(Iv_abc)
  Idc_pn (pu)/1 -> Signal Calculations/6(Idc_pn)
  PLL/1(Freq) -> [Freq]
  [Freq] -> Inner Current Loop/5(Freq)
  [Freq] -> DC Voltage Balance Control/4(Freq)
  [Freq] -> Signal Calculations/7(Freq)
  Clark Transformations/2(I_AB) -> Signal Calculations/2(I_AB)
  [U_AB] -> PLL/1(U_AB)
  PLL/3(Sin_Cos) -> [SinCos]
  [SinCos] -> Inner Current Loop/6(sin_cos)
  [SinCos] -> dq  Transformations/3(sin_cos)
  block_status/1 -> Outer Active-Reactive Power and Voltage Loop/10(block_status), Logical Operator1/1
  Signal Calculations/7(U_meas) -> Outer Active-Reactive Power and Voltage Loop/5(U_meas), [U_meas]
  Sum/1 -> Vref_abc/1
  Logical Operator1/1 -> Logical Operator2/2
  [Udc_meas] -> Inner Current Loop/3(Udc_meas)
  Signal Calculations/2(Mod_index) -> [Mod_index]
  DC Voltage Balance Control/1(dVref_abc) -> Sum/2
  Clark Transformations/4(Iv_AB) -> dq  Transformations/2(Iv_AB)
  Clark Transformations/3(Uf_AB) -> Signal Calculations/3(Uf_AB)
  Udref/1 -> Outer Active-Reactive Power and Voltage Loop/9(Udref)
  Bus Creator/1 -> m/1
  [U_meas] -> Bus Creator/1  "U_meas (pu)"
  [P_meas] -> Bus Creator/4  "P_meas (pu)"
  [Uf_meas] -> Bus Creator/2  "Uf_meas (pu)"
  [Iv_meas] -> Bus Creator/3  "Iv_meas (pu)"
  Outer Active-Reactive Power and Voltage Loop/2(Pref_ramped) -> [Pref_ramped]
  [Pref_ramped] -> Bus Creator/8  "Pref_ramped (pu)"
  Inner Current Loop/2(Vref_lim_AB) -> Signal Calculations/4(Vref_lim_AB)
  [Iv_dq] -> Bus Creator/10  "Iv_dq (pu)"
  DC Voltage Balance Control/2(Udc_0_mean) -> [Udc_0_mean]
  [Udc_0_mean] -> Bus Creator/12  "Udc_0_mean (pu)"
  Uabc (pu)/1 -> Clark Transformations/1("U_abc ")
  Iabc (pu)/1 -> Clark Transformations/2("I_abc ")
  Uf_abc (pu)/1 -> Clark Transformations/3("Uf_abc ")
  Iv_abc (pu)/1 -> Clark Transformations/4("Iv_abc "), [Iv_abc]
  [Q_meas] -> Bus Creator/5  "Q_meas (pu)"
  [Pdc_meas] -> Bus Creator/6  "Pdc_meas (pu)"
  [Iref_dq] -> Bus Creator/9  "Iref_dq (pu)"
  [Mod_index] -> Bus Creator/11  "Mod_index"
  Gain1/1 -> Bus Creator/7  "Udc_meas (pu)"
  [Udc_meas] -> Gain1/1

== system HVDC_VSC_1CPUcore_dcpl/SM_HVDC_VSC/VSC Controller (Station 2)/3-level firing pulse unit for TSB ==
  3 phase output frequency : Inport
  wt : Inport  Port=2
  Carriers Generator : Subsystem
  Demux3 : Demux  Outputs=3
  Gain5 : Gain  SaturateOnIntegerOverflow=on  OutDataTypeStr=Inherit: Same as input  ParamDataTypeStr=Inherit: Same as input
  Gain6 : Gain  SaturateOnIntegerOverflow=on  OutDataTypeStr=Inherit: Same as input  ParamDataTypeStr=Inherit: Same as input
  Mux3 : Mux  Inputs=12
  RTE Period Meter : rteventslib/Signal Attributes/RTE Period Meter  Period=off  Frequency=off  EdgeType=Rising edges  TOn=off  TOff=off  DutyCycle=on  DuringType=Calculation step  MinimumFrequency=0
  Subsystem1 : Subsystem
  Subsystem2 : Subsystem
  Subsystem6 : Subsystem
  duty : Outport
  wires:
  Mux3/1 -> RTE Period Meter/1
  Subsystem2/4(4) -> Mux3/12
  Subsystem2/3(3) -> Mux3/11
  Subsystem2/2(2) -> Mux3/10
  Subsystem2/1(1) -> Mux3/9
  Subsystem1/4(4) -> Mux3/8
  Subsystem1/3(3) -> Mux3/7
  Subsystem1/2(2) -> Mux3/6
  Subsystem1/1(1) -> Mux3/5
  Subsystem6/4(4) -> Mux3/4
  Subsystem6/3(3) -> Mux3/3
  Subsystem6/2(2) -> Mux3/2
  Subsystem6/1(1) -> Mux3/1
  Carriers Generator/2(C-) -> Gain6/1
  Carriers Generator/1(C+) -> Gain5/1
  Gain6/1 -> Subsystem1/3(c-), Subsystem2/3(c-), Subsystem6/3(c-)
  Gain5/1 -> Subsystem1/2(c+), Subsystem2/2(c+), Subsystem6/2(c+)
  wt/1 -> Carriers Generator/1(theta)
  Demux3/1 -> Subsystem6/1(in)
  Demux3/2 -> Subsystem1/1(in)
  Demux3/3 -> Subsystem2/1(in)
  3 phase output frequency/1 -> Demux3/1
  RTE Period Meter/1 -> duty/1

== system HVDC_VSC_1CPUcore_dcpl/SM_HVDC_VSC/VSC Controller (Station 2)/Anti-aliasing Filters ==
  note: Low-pass filter
  note: Filtering
  "Uabc " : Inport  PortDimensions=3
  "Iabc " : Inport  Port=2  PortDimensions=3
  "Uf_abc  " : Inport  Port=3  PortDimensions=3
  "Iv_abc " : Inport  Port=4  PortDimensions=3
  "Udc_pn  " : Inport  Port=5
  "Idc_pn " : Inport  Port=6
  2nd-Order Filter{1..9} (9 alike) : powerlib_extras/Discrete  Control Blocks/Discrete  2nd-Order Filter  FilterType=Lowpass  Fo=f0_aa  Zeta=zeta  Ts=Ts_Control  Initialize=off  Vac_Init=[0.8 -25 60]  Vdc_Init=-0.4  PlotResponse=off  param1=[1 2000 0.2]
  2nd-Order f0_aa {,1..6} (7 alike) : powerlib_extras/Discrete  Control Blocks/Discrete  2nd-Order Filter  FilterType=Lowpass  Fo=f0_aa  Zeta=zeta  Ts=Ts_Control  Initialize=off  Vac_Init=[0.8 -25 60]  Vdc_Init=-0.4  PlotResponse=off  param1=[1 2000 0.2]
  Demux{,1..3} (4 alike) : Demux  Outputs=3
  Demux4 : Demux  Outputs=2
  Demux5 : Demux  Outputs=2
  Mux{,1..3} (4 alike) : Mux  Inputs=3
  Mux4 : Mux  Inputs=2
  Mux5 : Mux  Inputs=2
  Uabc : Outport
  Iabc : Outport  Port=2
  Uf_abc : Outport  Port=3
  " Iv_abc" : Outport  Port=4
  "Udc_pn " : Outport  Port=5
  " Idc_pn" : Outport  Port=6
  wires:
  "Udc_pn  "/1 -> Demux5/1
  Demux5/2 -> 2nd-Order f0_aa 1/1
  Demux5/1 -> "2nd-Order f0_aa "/1
  "Idc_pn "/1 -> Demux4/1
  Demux4/2 -> 2nd-Order f0_aa 3/1
  Demux4/1 -> 2nd-Order f0_aa 2/1
  Mux5/1 -> "Udc_pn "/1
  2nd-Order f0_aa 1/1 -> Mux5/2
  "2nd-Order f0_aa "/1 -> Mux5/1
  Mux4/1 -> " Idc_pn"/1
  2nd-Order f0_aa 3/1 -> Mux4/2
  2nd-Order f0_aa 2/1 -> Mux4/1
  2nd-Order Filter9/1 -> Mux/1
  Demux/1 -> 2nd-Order Filter9/1
  "Iabc "/1 -> Demux3/1
  Demux3/1 -> 2nd-Order f0_aa 4/1
  2nd-Order f0_aa 4/1 -> Mux3/1
  2nd-Order f0_aa 5/1 -> Mux3/2
  2nd-Order f0_aa 6/1 -> Mux3/3
  Demux3/3 -> 2nd-Order f0_aa 6/1
  Demux3/2 -> 2nd-Order f0_aa 5/1
  Mux3/1 -> Iabc/1
  "Uabc "/1 -> Demux2/1
  Demux2/1 -> 2nd-Order Filter6/1
  2nd-Order Filter6/1 -> Mux2/1
  2nd-Order Filter7/1 -> Mux2/2
  2nd-Order Filter8/1 -> Mux2/3
  Demux2/3 -> 2nd-Order Filter8/1
  Demux2/2 -> 2nd-Order Filter7/1
  Mux2/1 -> Uabc/1
  "Iv_abc "/1 -> Demux/1
  Mux/1 -> " Iv_abc"/1
  2nd-Order Filter1/1 -> Mux/2
  2nd-Order Filter2/1 -> Mux/3
  Demux/3 -> 2nd-Order Filter2/1
  Demux/2 -> 2nd-Order Filter1/1
  "Uf_abc  "/1 -> Demux1/1
  Demux1/1 -> 2nd-Order Filter3/1
  2nd-Order Filter3/1 -> Mux1/1
  2nd-Order Filter4/1 -> Mux1/2
  2nd-Order Filter5/1 -> Mux1/3
  Demux1/3 -> 2nd-Order Filter5/1
  Demux1/2 -> 2nd-Order Filter4/1
  Mux1/1 -> Uf_abc/1

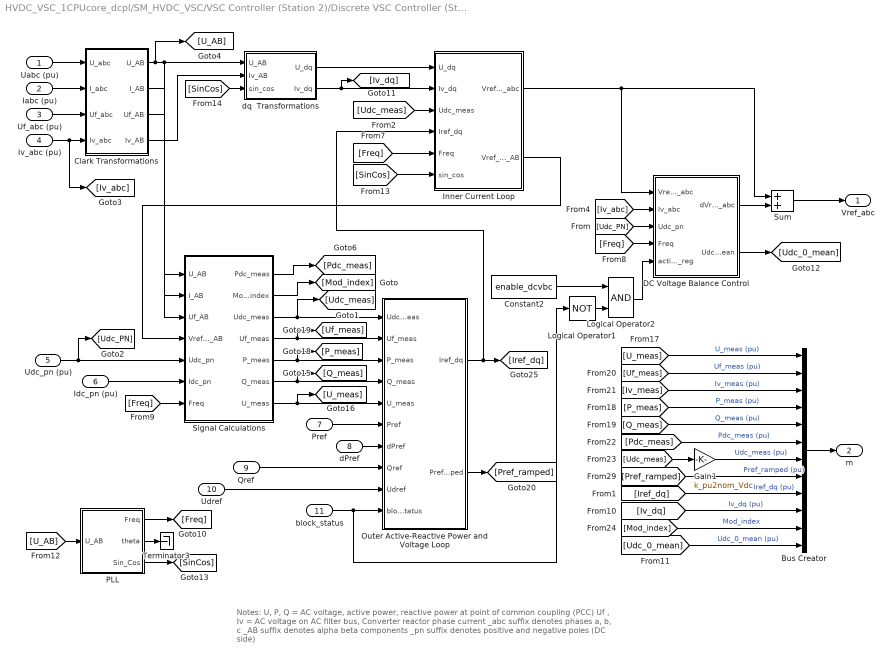
== system HVDC_VSC_1CPUcore_dcpl/SM_HVDC_VSC/VSC Controller (Station 2)/Discrete VSC Controller (Station 2) ==
  note: Notes:
      | U, P, Q = AC voltage, active power, reactive power at point of common coupling (PCC)
      | Uf , Iv  = AC voltage on AC filter bus, Converter reactor phase current
      | _abc suffix denotes phases a, b, c
      | _AB  suffix denotes alpha beta components
      | _pn  suffix denotes positive and negative poles (DC side)
  Uabc (pu) : Inport
  Iabc (pu) : Inport  Port=2
  Uf_abc (pu) : Inport  Port=3
  Iv_abc (pu) : Inport  Port=4
  Udc_pn (pu) : Inport  Port=5
  Idc_pn (pu) : Inport  Port=6
  Pref : Inport  Port=7
  dPref : Inport  Port=8
  Qref : Inport  Port=9
  Udref : Inport  Port=10
  block_status : Inport  Port=11
  Bus Creator : BusCreator  Inputs=12
  Clark Transformations : Subsystem
  Constant2 : Constant  Value=enable_dcvbc
  DC Voltage Balance Control : Subsystem
  Gain1 : Gain  Gain=k_pu2nom_Vdc  SaturateOnIntegerOverflow=on  OutDataTypeStr=Inherit: Same as input  ParamDataTypeStr=Inherit: Same as input
  Inner Current Loop : Subsystem
  Logical Operator1 : Logic  Operator=NOT  Inputs=1  AllPortsSameDT=off
  Logical Operator2 : Logic  AllPortsSameDT=off
  Outer Active-Reactive Power and Voltage Loop : Subsystem
  PLL : Subsystem  AncestorBlock=|  mask(Discrete 3-phase PLL){Fmin=f_min_pll, Par_Init=[0   60], ParK=[Kp_pll  Ki_pll], Ts=Ts_Control}
      | powerlib_extras/Discrete 
      | Control Blocks/Discrete
      | 3-phase PLL
      mask prompts: Fmin "Minimum frequency (Hz):"; Par_Init "Initial inputs:[ Phase(degrees)   Frequency(Hz) ]"; ParK "Regulator gains [ Kp  Ki ]"; Ts "Sample time:"
      mask help:
      | This Phase Locked Loop (PLL) system can be used  to synchronize on a set of variable frequency, three-phase sinusoidal signals.
      |
      | Input 1: Vector containing the normalized
      |              three-phase signals [Va Vb Vc]
      | Output 1:  Measured frequency (Hz) = w/(2pi)
      | Output 2:  Ramp w.t   varying between  0 and 2*pi,
      | synchronized on zero crossings of the fundamental (positive-sequence) of phase A.
      | Output 3: Vector [sin(wt) cos(wt)]
      mask init:
      | Kp=ParK(1);
      | Ki=ParK(2);
      | Phase_Init=Par_Init(1);
      | Finit=Par_Init(2);
  Signal Calculations : Subsystem
  Sum : Sum  SaturateOnIntegerOverflow=on
  Terminator3 : Terminator
  dq  Transformations : Subsystem
  Vref_abc : Outport
  m : Outport  Port=2
  wires:
  Outer Active-Reactive Power and Voltage Loop/1(Iref_dq) -> Inner Current Loop/4(Iref_dq), [Iref_dq]
  dq  Transformations/2(Iv_dq) -> Inner Current Loop/2(Iv_dq), [Iv_dq]
  Inner Current Loop/1(Vref_lim_abc) -> Sum/1, DC Voltage Balance Control/1(Vref_lim_abc)
  dq  Transformations/1(U_dq) -> Inner Current Loop/1(U_dq)
  Signal Calculations/3(Udc_meas) -> Outer Active-Reactive Power and Voltage Loop/1(Udc_meas), [Udc_meas]
  Signal Calculations/4(Uf_meas) -> Outer Active-Reactive Power and Voltage Loop/2(Uf_meas), [Uf_meas]
  Signal Calculations/6(Q_meas) -> Outer Active-Reactive Power and Voltage Loop/4(Q_meas), [Q_meas]
  Signal Calculations/5(P_meas) -> Outer Active-Reactive Power and Voltage Loop/3(P_meas), [P_meas]
  Clark Transformations/1(U_AB) -> dq  Transformations/1(U_AB), Signal Calculations/1(U_AB), [U_AB]
  Signal Calculations/1(Pdc_meas) -> [Pdc_meas]
  Constant2/1 -> Logical Operator2/1
  Pref/1 -> Outer Active-Reactive Power and Voltage Loop/6(Pref)
  dPref/1 -> Outer Active-Reactive Power and Voltage Loop/7(dPref)
  Qref/1 -> Outer Active-Reactive Power and Voltage Loop/8(Qref)
  PLL/2(theta) -> Terminator3/1
  Logical Operator2/1 -> DC Voltage Balance Control/5(activate_reg)
  [Udc_PN] -> DC Voltage Balance Control/3(Udc_pn)
  Udc_pn (pu)/1 -> Signal Calculations/5(Udc_pn), [Udc_PN]
  [Iv_abc] -> DC Voltage Balance Control/2(Iv_abc)
  Idc_pn (pu)/1 -> Signal Calculations/6(Idc_pn)
  PLL/1(Freq) -> [Freq]
  [Freq] -> Inner Current Loop/5(Freq)
  [Freq] -> DC Voltage Balance Control/4(Freq)
  [Freq] -> Signal Calculations/7(Freq)
  Clark Transformations/2(I_AB) -> Signal Calculations/2(I_AB)
  [U_AB] -> PLL/1(U_AB)
  PLL/3(Sin_Cos) -> [SinCos]
  [SinCos] -> Inner Current Loop/6(sin_cos)
  [SinCos] -> dq  Transformations/3(sin_cos)
  block_status/1 -> Outer Active-Reactive Power and Voltage Loop/10(block_status), Logical Operator1/1
  Signal Calculations/7(U_meas) -> Outer Active-Reactive Power and Voltage Loop/5(U_meas), [U_meas]
  Sum/1 -> Vref_abc/1
  Logical Operator1/1 -> Logical Operator2/2
  [Udc_meas] -> Inner Current Loop/3(Udc_meas)
  Signal Calculations/2(Mod_index) -> [Mod_index]
  DC Voltage Balance Control/1(dVref_abc) -> Sum/2
  Clark Transformations/4(Iv_AB) -> dq  Transformations/2(Iv_AB)
  Clark Transformations/3(Uf_AB) -> Signal Calculations/3(Uf_AB)
  Udref/1 -> Outer Active-Reactive Power and Voltage Loop/9(Udref)
  Bus Creator/1 -> m/1
  [U_meas] -> Bus Creator/1  "U_meas (pu)"
  [P_meas] -> Bus Creator/4  "P_meas (pu)"
  [Uf_meas] -> Bus Creator/2  "Uf_meas (pu)"
  [Iv_meas] -> Bus Creator/3  "Iv_meas (pu)"
  Outer Active-Reactive Power and Voltage Loop/2(Pref_ramped) -> [Pref_ramped]
  [Pref_ramped] -> Bus Creator/8  "Pref_ramped (pu)"
  Inner Current Loop/2(Vref_lim_AB) -> Signal Calculations/4(Vref_lim_AB)
  [Iv_dq] -> Bus Creator/10  "Iv_dq (pu)"
  DC Voltage Balance Control/2(Udc_0_mean) -> [Udc_0_mean]
  [Udc_0_mean] -> Bus Creator/12  "Udc_0_mean (pu)"
  Uabc (pu)/1 -> Clark Transformations/1("U_abc ")
  Iabc (pu)/1 -> Clark Transformations/2("I_abc ")
  Uf_abc (pu)/1 -> Clark Transformations/3("Uf_abc ")
  Iv_abc (pu)/1 -> Clark Transformations/4("Iv_abc "), [Iv_abc]
  [Q_meas] -> Bus Creator/5  "Q_meas (pu)"
  [Pdc_meas] -> Bus Creator/6  "Pdc_meas (pu)"
  [Iref_dq] -> Bus Creator/9  "Iref_dq (pu)"
  [Mod_index] -> Bus Creator/11  "Mod_index"
  Gain1/1 -> Bus Creator/7  "Udc_meas (pu)"
  [Udc_meas] -> Gain1/1

== system HVDC_VSC_1CPUcore_dcpl/SM_HVDC_VSC/WSCC System 1/Bus_1 16.5 KV ==
  Kv : Gain  Gain=Ki  SaturateOnIntegerOverflow=on  OutDataTypeStr=Inherit: Same as input  ParamDataTypeStr=Inherit: Same as input
  Kv1 : Gain  Gain=Kv  SaturateOnIntegerOverflow=on  OutDataTypeStr=Inherit: Same as input  ParamDataTypeStr=Inherit: Same as input
  Mode I : spsVIMeasurementModel/Complex
  Mode V : spsVIMeasurementModel/Complex
  Model : spsVIMeasurementModel/VI_phase  SystemSampleTime=-1
  A : PMIOPort  Port=1  Side=Left
  B : PMIOPort  Port=2  Side=Left
  C : PMIOPort  Port=3  Side=Left
  a : PMIOPort  Port=4  Side=Right
  b : PMIOPort  Port=5  Side=Right
  c : PMIOPort  Port=6  Side=Right
  tag scope: Iabc_1=global, Vabc_1=global
  wires:
  Model/2 -> Kv/1
  Model/1 -> Kv1/1
  Kv/1 -> Mode I/1
  Kv1/1 -> Mode V/1
  Mode I/1 -> [Iabc_1]
  Mode V/1 -> [Vabc_1]
  connections:
  Model/RConn3 -- c/RConn1
  Model/RConn1 -- a/RConn1
  Model/RConn2 -- b/RConn1
  Model/LConn3 -- C/RConn1
  Model/LConn1 -- A/RConn1
  Model/LConn2 -- B/RConn1

== system HVDC_VSC_1CPUcore_dcpl/SM_HVDC_VSC/WSCC System 1/Bus_2 18 KV ==
  Kv : Gain  Gain=Ki  SaturateOnIntegerOverflow=on  OutDataTypeStr=Inherit: Same as input  ParamDataTypeStr=Inherit: Same as input
  Kv1 : Gain  Gain=Kv  SaturateOnIntegerOverflow=on  OutDataTypeStr=Inherit: Same as input  ParamDataTypeStr=Inherit: Same as input
  Mode I : spsVIMeasurementModel/Complex
  Mode V : spsVIMeasurementModel/Complex
  Model : spsVIMeasurementModel/VI_phase  SystemSampleTime=-1
  A : PMIOPort  Port=1  Side=Left
  B : PMIOPort  Port=2  Side=Left
  C : PMIOPort  Port=3  Side=Left
  a : PMIOPort  Port=4  Side=Right
  b : PMIOPort  Port=5  Side=Right
  c : PMIOPort  Port=6  Side=Right
  tag scope: Iabc_2=global, Vabc_2=global
  wires:
  Model/2 -> Kv/1
  Model/1 -> Kv1/1
  Kv/1 -> Mode I/1
  Kv1/1 -> Mode V/1
  Mode I/1 -> [Iabc_2]
  Mode V/1 -> [Vabc_2]
  connections:
  Model/RConn3 -- c/RConn1
  Model/RConn1 -- a/RConn1
  Model/RConn2 -- b/RConn1
  Model/LConn3 -- C/RConn1
  Model/LConn1 -- A/RConn1
  Model/LConn2 -- B/RConn1

== system HVDC_VSC_1CPUcore_dcpl/SM_HVDC_VSC/WSCC System 1/Bus_3 13.8 KV ==
  Kv : Gain  Gain=Ki  SaturateOnIntegerOverflow=on  OutDataTypeStr=Inherit: Same as input  ParamDataTypeStr=Inherit: Same as input
  Kv1 : Gain  Gain=Kv  SaturateOnIntegerOverflow=on  OutDataTypeStr=Inherit: Same as input  ParamDataTypeStr=Inherit: Same as input
  Mode I : spsVIMeasurementModel/Complex
  Mode V : spsVIMeasurementModel/Complex
  Model : spsVIMeasurementModel/VI_phase  SystemSampleTime=-1
  A : PMIOPort  Port=1  Side=Left
  B : PMIOPort  Port=2  Side=Left
  C : PMIOPort  Port=3  Side=Left
  a : PMIOPort  Port=4  Side=Right
  b : PMIOPort  Port=5  Side=Right
  c : PMIOPort  Port=6  Side=Right
  tag scope: Iabc_3=global, Vabc_3=global
  wires:
  Model/2 -> Kv/1
  Model/1 -> Kv1/1
  Kv/1 -> Mode I/1
  Kv1/1 -> Mode V/1
  Mode I/1 -> [Iabc_3]
  Mode V/1 -> [Vabc_3]
  connections:
  Model/RConn3 -- c/RConn1
  Model/RConn1 -- a/RConn1
  Model/RConn2 -- b/RConn1
  Model/LConn3 -- C/RConn1
  Model/LConn1 -- A/RConn1
  Model/LConn2 -- B/RConn1
